simulink model "Water_Tank_Temperature"  (R2024b)
settings: Solver=VariableStepAuto  StartTime=0.0  StopTime=100  RelTol=1e-3
settings Model: Creator=Umesh Reddy K  LastModifiedBy=Umesh Reddy K

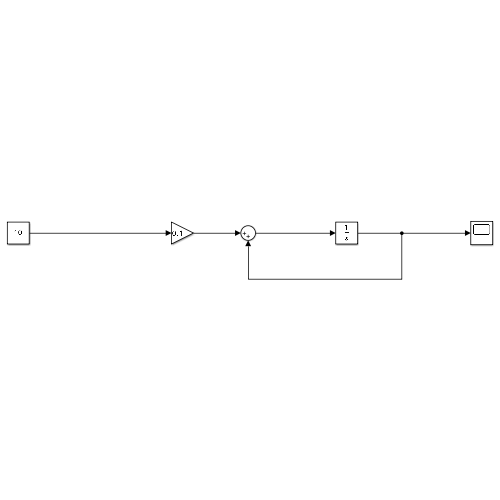
[thumbnail: Simulink's stored preview of the top-level diagram]
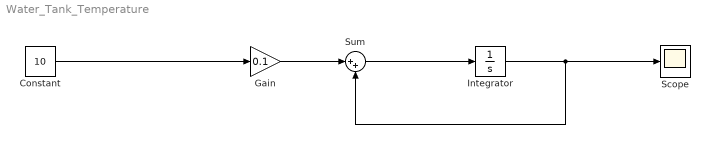
== system Water_Tank_Temperature ==
  Constant : Constant  Value=10
  Gain : Gain  Gain=0.1
  Integrator : Integrator  InitialCondition=20
  Scope : Scope
  Sum : Sum  Inputs=|++
  wires:
  Constant/1 -> Gain/1
  Gain/1 -> Sum/1
  Sum/1 -> Integrator/1
  Integrator/1 -> Sum/2, Scope/1
